simulink model "SuspensionSimulink"  (R2025b)
settings: Solver=VariableStepAuto  StartTime=0.0  StopTime=10.0  RelTol=1e-3
values from neighbouring files (symbols this model uses):
  b1 = 1000    [Suspension.m]    (also in parametrosSuspencion - copia.m; practica2A_ValeriaSinaiLaraRojas.m)
  f = 0    [Suspension.m]    (also in parametrosSuspencion - copia.m; practica2A_ValeriaSinaiLaraRojas.m)
  k1 = 16182    [Suspension.m]    (also in parametrosSuspencion - copia.m; practica2A_ValeriaSinaiLaraRojas.m)
  k2 = 19000    [Suspension.m]    (also in parametrosSuspencion - copia.m; practica2A_ValeriaSinaiLaraRojas.m)
  m1 = 290    [Suspension.m]    (also in parametrosSuspencion - copia.m; practica2A_ValeriaSinaiLaraRojas.m)
  m2 = 59    [Suspension.m]    (also in parametrosSuspencion - copia.m; practica2A_ValeriaSinaiLaraRojas.m)
  z1 = @(t) 0.05 * sin(0.5 * pi * t)    [practica2A_ValeriaSinaiLaraRojas.m]
settings Model: Creator=Cecilia  LastModifiedBy=Cecilia

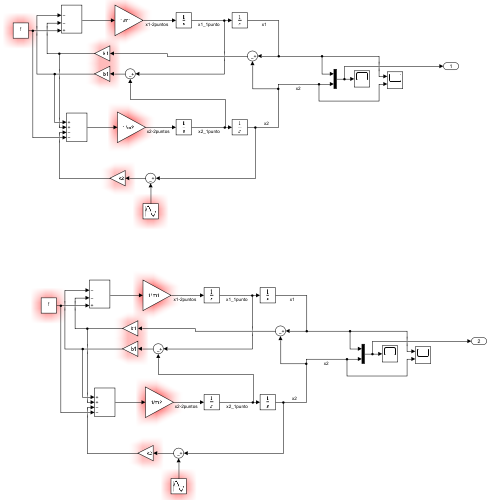
[thumbnail: Simulink's stored preview of the top-level diagram]
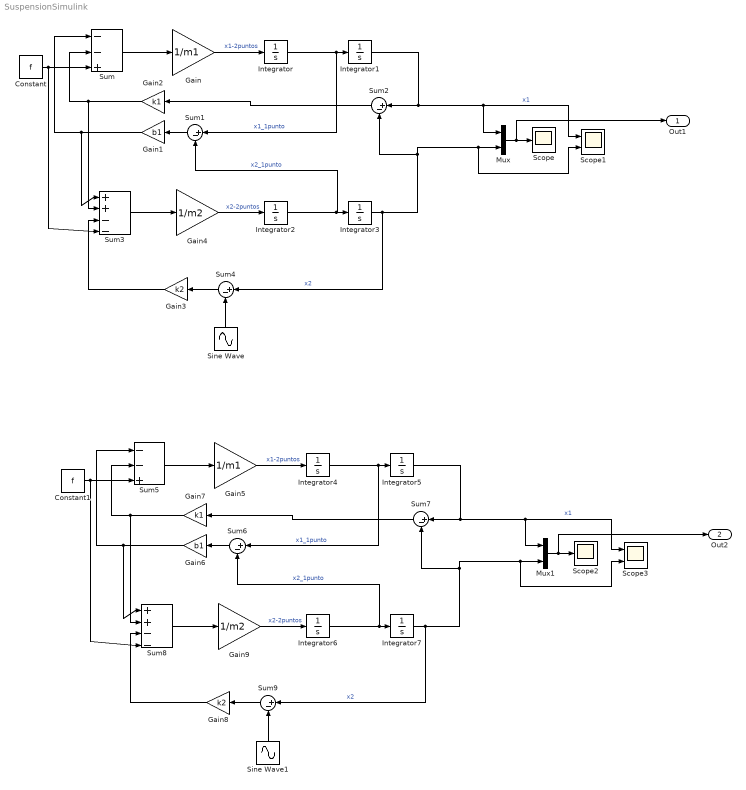
== system SuspensionSimulink ==
  Constant : Constant  Value=f
  Constant1 : Constant  Value=f
  Gain : Gain  Gain=1/m1
  Gain1 : Gain  Gain=b1
  Gain2 : Gain  Gain=k1
  Gain3 : Gain  Gain=k2
  Gain4 : Gain  Gain=1/m2
  Gain5 : Gain  Gain=1/m1
  Gain6 : Gain  Gain=b1
  Gain7 : Gain  Gain=k1
  Gain8 : Gain  Gain=k2
  Gain9 : Gain  Gain=1/m2
  Integrator{,1..7} (8 alike) : Integrator
  Mux : Mux  Inputs=2
  Mux1 : Mux  Inputs=2
  Scope : Scope
      settings: ActiveDisplayYMinimum=-0.0081004107203286064  ActiveDisplayYMaximum=0.013153550265285642
  Scope1 : Scope  NumInputPorts=2
      settings: ActiveDisplayYMinimum=-0.070244155943805647  ActiveDisplayYMaximum=0.080568186773229425
  Scope2 : Scope
      settings: ActiveDisplayYMinimum=-0.0081004107203286064  ActiveDisplayYMaximum=0.013153550265285642  DataLoggingVariableName=ScopeData2
  Scope3 : Scope  NumInputPorts=2
      settings: ActiveDisplayYMinimum=-0.070244155943805647  ActiveDisplayYMaximum=0.080568186773229425  DataLoggingVariableName=ScopeData3
  Sine Wave : Sin  Amplitude=.05  Frequency=z1  SampleTime=0
  Sine Wave1 : Sin  Amplitude=.05  Frequency=z1  SampleTime=0
  Sum : Sum  Inputs=|--+
  Sum{1..2,4,6..7,9} (6 alike) : Sum  Inputs=|+-
  Sum3 : Sum  Inputs=|++--
  Sum5 : Sum  Inputs=|--+
  Sum8 : Sum  Inputs=|++--
  Out1 : Outport
  Out2 : Outport  Port=2
  wires:
  Sum3/1 -> Gain4/1
  Sum2/1 -> Gain2/1
  Sum4/1 -> Gain3/1
  Integrator2/1 -> Sum1/2, Integrator3/1  "x2_1punto"
  Sum1/1 -> Gain1/1
  Gain2/1 -> Sum3/2, Sum/2
  Gain1/1 -> Sum3/1, Sum/1
  Mux/1 -> Out1/1, Scope/1
  Sine Wave/1 -> Sum4/2
  Gain4/1 -> Integrator2/1  "x2-2puntos"
  Integrator3/1 -> Sum4/1, Scope1/2, Mux/2, Sum2/2  "x2"
  Constant/1 -> Sum3/4, Sum/3
  Integrator/1 -> Sum1/1, Integrator1/1  "x1_1punto"
  Gain3/1 -> Sum3/3
  Gain/1 -> Integrator/1  "x1-2puntos"
  Integrator1/1 -> Scope1/1, Mux/1, Sum2/1  "x1"
  Sum/1 -> Gain/1
  Sum8/1 -> Gain9/1
  Sum7/1 -> Gain7/1
  Sum9/1 -> Gain8/1
  Integrator6/1 -> Sum6/2, Integrator7/1  "x2_1punto"
  Sum6/1 -> Gain6/1
  Gain7/1 -> Sum8/2, Sum5/2
  Gain6/1 -> Sum8/1, Sum5/1
  Mux1/1 -> Out2/1, Scope2/1
  Sine Wave1/1 -> Sum9/2
  Gain9/1 -> Integrator6/1  "x2-2puntos"
  Integrator7/1 -> Sum9/1, Scope3/2, Mux1/2, Sum7/2  "x2"
  Constant1/1 -> Sum8/4, Sum5/3
  Integrator4/1 -> Sum6/1, Integrator5/1  "x1_1punto"
  Gain8/1 -> Sum8/3
  Gain5/1 -> Integrator4/1  "x1-2puntos"
  Integrator5/1 -> Scope3/1, Mux1/1, Sum7/1  "x1"
  Sum5/1 -> Gain5/1
